simulink model "B4_quadcopter_model_discrete"  (R2021b)
settings: Solver=VariableStepAuto  StartTime=0.0  StopTime=10  FixedStep=0.002  RelTol=1e-3
values from neighbouring files (symbols this model uses):
  coef_sim_1 = tf_des_d.Denominator{1}(2)    [A11_setup_script_pprz.m]    (also in A1_setup_script.m; A6_slow_actuator.m)
  coef_sim_2 = tf_des_d.Numerator{1}(2)    [A11_setup_script_pprz.m]    (also in A1_setup_script.m; A6_slow_actuator.m)
  doublet_mag = - 0.15    (= -0.15)    [A11_setup_script_pprz.m]    (also in A1_setup_script.m)
  doublet_time = 6    [A11_setup_script_pprz.m]    (also in A1_setup_script.m)
  f_8 = 1    [A11_setup_script_pprz.m]    (also in A1_setup_script.m)
  FILT_CUTOFF = 2*pi*5    (= 31.4159265359)    [A11_setup_script_pprz.m]    (also in A1_setup_script.m)
  FILTER = 1    [A11_setup_script_pprz.m]    (also in A1_setup_script.m)
  G1 = inv(I)*G1_r    [A10_simple_plant.m]    (also in A11_setup_script_pprz.m = G1/scale; A1_setup_script.m = [G1;G1_T])
  G1_simple = inv(I)*G1_r_simple    [A1_setup_script.m]
  G2 = G2/scale    [A11_setup_script_pprz.m]    (also in A1_setup_script.m = (1/sampling_time)*inv(I)*(G2_r))
  h_plate = 0.3    [A11_setup_script_pprz.m]    (also in A1_setup_script.m = 0.16)
  I = eye(3,3)    [A10_simple_plant.m]    (also in A11_setup_script_pprz.m; A1_setup_script.m; A2_B_matrix_generation_symbolic.m = [Ixx 0 0; A3_B_matrix_generation_symbolic_cascaded.m = [Ixx 0 0)
  Iyy = 0.0008    [A11_setup_script_pprz.m]    (also in A1_setup_script.m = 0.0015)
  Izz = 0.000498    [A11_setup_script_pprz.m]    (also in A1_setup_script.m = 0.00015)
  K = 7    [A11_setup_script_pprz.m]    (also in A1_setup_script.m = 10)
  K_act = 50    [A10_simple_plant.m]    (also in A11_setup_script_pprz.m = 20; A1_setup_script.m = 20)
  K_act_outer = diag([K K K_act])    [A1_setup_script.m]
  K_d = 15    [A11_setup_script_pprz.m]    (also in A1_setup_script.m = 25)
  K_dd = K_act    (= 20)    [A11_setup_script_pprz.m]    (also in A1_setup_script.m)
  K_dyn = K    (= 10)    [A1_setup_script.m]
  K_ec = 50    [A11_setup_script_pprz.m]    (also in A1_setup_script.m = 251)
  K_ec_d = 13    [A11_setup_script_pprz.m]    (also in A1_setup_script.m = 25)
  K_ec_d_u = 1.5    [A11_setup_script_pprz.m]    (also in A1_setup_script.m = 5)
  K_ec_d_v = 1.5    [A11_setup_script_pprz.m]    (also in A1_setup_script.m = 5)
  K_ec_d_w = 1.5    [A11_setup_script_pprz.m]    (also in A1_setup_script.m = 5)
  K_ec_dd = 9    [A11_setup_script_pprz.m]    (also in A1_setup_script.m = 45)
  K_ec_i = 0    [A11_setup_script_pprz.m]    (also in A1_setup_script.m = 380)
  K_ec_u = 1.5    [A11_setup_script_pprz.m]    (also in A1_setup_script.m = 5)
  K_ec_v = 1.5    [A11_setup_script_pprz.m]    (also in A1_setup_script.m = 5)
  K_ec_w = 1.5    [A11_setup_script_pprz.m]    (also in A1_setup_script.m = 5)
  K_t = 0.0005    [A10_simple_plant.m]    (also in A11_setup_script_pprz.m = 6.557e-08; A1_setup_script.m = 6.557e-08)
  K_u = 1.0    (= 1)    [A11_setup_script_pprz.m]    (also in A1_setup_script.m = 1.5)
  K_u_d = 2.5    [A11_setup_script_pprz.m]    (also in A1_setup_script.m = 7)
  K_u_dd = K    (= 10)    [A1_setup_script.m]
  K_v = 1.0    (= 1)    [A11_setup_script_pprz.m]    (also in A1_setup_script.m = 1.5)
  K_v_d = 2.5    [A11_setup_script_pprz.m]    (also in A1_setup_script.m = 7)
  K_v_dd = K    (= 10)    [A1_setup_script.m]
  K_w = 1.0    (= 1)    [A11_setup_script_pprz.m]    (also in A1_setup_script.m = 4.5)
  K_w_d = 2.5    [A11_setup_script_pprz.m]    (also in A1_setup_script.m = 7)
  K_w_dd = K    (= 10)    [A1_setup_script.m]
  l_plate = 0.1    [A11_setup_script_pprz.m]    (also in A1_setup_script.m = 0.11)
  m = 0.4    [A10_simple_plant.m]    (also in A11_setup_script_pprz.m; A1_setup_script.m)
  NOISE = 0    [A11_setup_script_pprz.m]    (also in A1_setup_script.m)
  NOISE_ACC = 0.00005    (= 5e-05)    [A11_setup_script_pprz.m]    (also in A1_setup_script.m)
  NOISE_GYRO = 0.00005    (= 5e-05)    [A11_setup_script_pprz.m]    (also in A1_setup_script.m)
  NOISE_RPM = 200    [A11_setup_script_pprz.m]    (also in A1_setup_script.m)
  omega_act = 50    [A6_slow_actuator.m]
  omega_des = 20.00    (= 20)    [A11_setup_script_pprz.m]    (also in A1_setup_script.m; A6_slow_actuator.m = 49)
  sampling_time = 1/frequency    (= 0.002)    [A11_setup_script_pprz.m]    (also in A12_sim_multi_run.m; A1_setup_script.m; A6_slow_actuator.m)
  scale_8 = 1.6    [A11_setup_script_pprz.m]    (also in A1_setup_script.m)
  start_8 = 2    [A11_setup_script_pprz.m]    (also in A1_setup_script.m)
  start_time = 2    [A11_setup_script_pprz.m]    (also in A1_setup_script.m = 1)
  t_8 = 10    [A11_setup_script_pprz.m]    (also in A1_setup_script.m)
  w_plate = 0.3    [A11_setup_script_pprz.m]    (also in A1_setup_script.m = 0.36)
undefined symbols (not defined in the file or in its folder): DiscIntNeverNeededParam, K_ec_d_p, K_ec_d_q, K_ec_d_r, K_ec_dd_p, K_ec_dd_q, K_ec_dd_r, K_ec_i_u, K_ec_i_v, K_ec_i_w, K_ec_p, K_ec_q, K_ec_r, K_p, K_p_d, K_p_dd, K_q, K_q_d, K_q_dd, K_r, K_r_d, K_r_dd
libraries: simulink x44, cstblocks x37, dspinverses x26, dspmathops x9, dspstat3 x9, aerolibutil x9, sharedutil x3, aerolibanim x1
(part 7 of 13)

== system B4_quadcopter_model_discrete/Discrete Model - Complementary Filtering/Discrete INDI Controller Cascaded w// Actuator Compensation/ERROR CONTROLLER VELOCITY ==
  Vx_ref : Inport
  Vy_ref : Inport  Port=2
  Vz_ref : Inport  Port=3
  X_ref : Inport  Port=4
  Y_ref : Inport  Port=5
  Z_ref : Inport  Port=6
  Gain : Gain  Gain=K_ec_u
  Gain1 : Gain  Gain=K_ec_d_u
  Gain2 : Gain  Gain=K_ec_v
  Gain3 : Gain  Gain=K_ec_d_v
  Gain4 : Gain  Gain=K_ec_v
  Gain5 : Gain  Gain=K_ec_d_v
  Sum{,3,5..8} (6 alike) : Sum  Inputs=|+-
  Sum1 : Sum  Inputs=|++
  Sum2 : Sum  Inputs=|++
  Sum4 : Sum  Inputs=|++
  Ax_ec : Outport
  Ay_ec : Outport  Port=2
  Az_ec : Outport  Port=3
  wires:
  [Vz] -> Sum6/2
  Sum1/1 -> Ax_ec/1
  Sum2/1 -> Ay_ec/1
  Vy_ref/1 -> Sum3/1
  Vx_ref/1 -> Sum/1
  [Vy] -> Sum3/2
  Vz_ref/1 -> Sum6/1
  Sum/1 -> Gain1/1  "Vx_error"
  Sum4/1 -> Az_ec/1
  [Vx] -> Sum/2
  [x] -> Sum5/2
  X_ref/1 -> Sum5/1
  Sum5/1 -> Gain/1
  Gain1/1 -> Sum1/1
  Gain/1 -> Sum1/2
  Gain3/1 -> Sum2/1
  Sum3/1 -> Gain3/1  "Vy_error"
  Gain5/1 -> Sum4/1
  Sum6/1 -> Gain5/1  "Vz_error"
  Y_ref/1 -> Sum7/1
  [y] -> Sum7/2
  Sum7/1 -> Gain2/1
  Z_ref/1 -> Sum8/1
  [z] -> Sum8/2
  Sum8/1 -> Gain4/1
  Gain4/1 -> Sum4/2
  Gain2/1 -> Sum2/2

== system B4_quadcopter_model_discrete/Discrete Model - Complementary Filtering/Discrete INDI Controller Cascaded w// Actuator Compensation/INTERNAL REFERENCE MODEL ATTITUDE ==
  phi_cmd : Inport
  theta_cmd : Inport  Port=2
  psi_cmd : Inport  Port=3
  Discrete-Time Integrator{,1..8} (9 alike) : DiscreteIntegrator  SampleTime=sampling_time  ICPrevOutput=DiscIntNeverNeededParam  ICPrevScaledInput=DiscIntNeverNeededParam
  Gain1 : Gain  Gain=K
  Gain2 : Gain  Gain=K_dd
  Gain3 : Gain  Gain=K
  Gain4 : Gain  Gain=K_d
  Gain5 : Gain  Gain=K_d
  Gain6 : Gain  Gain=K_d
  Gain7 : Gain  Gain=K
  Gain8 : Gain  Gain=K_dd
  Gain9 : Gain  Gain=K_dd
  MATLAB Function1 : MATLAB Function  TreatAsAtomicUnit=on
  Scope : Scope  NumInputPorts=2
  Sum{1..4,11,16,20..22} (9 alike) : Sum  Inputs=|+-
  body rates to euler rates : Subsystem
  euler rates to body rates : Subsystem
  pdd_ref : Outport
  qdd_ref : Outport  Port=2
  rdd_ref : Outport  Port=3
  pd_ref : Outport  Port=4
  qd_ref : Outport  Port=5
  rd_ref : Outport  Port=6
  p_ref : Outport  Port=7
  q_ref : Outport  Port=8
  r_ref : Outport  Port=9
  phi_ref : Outport  Port=10
  theta_ref : Outport  Port=11
  psi_ref : Outport  Port=12
  tag scope: p_ref=global, phi_ref=global, psi_ref=global, q_ref=global, r_ref=global, theta_ref=global
  wires:
  Discrete-Time Integrator1/1 -> [theta_ref], theta_ref/1, Sum11/2  "theta_ref"
  Discrete-Time Integrator8/1 -> Sum4/2, Discrete-Time Integrator5/1, rd_ref/1  "rd_ref"
  Discrete-Time Integrator3/1 -> [p_ref], p_ref/1, body rates to euler rates/1(p), Sum21/2  "p_ref"
  Discrete-Time Integrator5/1 -> [r_ref], r_ref/1, body rates to euler rates/3(r), Sum22/2  "r_ref"
  Discrete-Time Integrator4/1 -> Scope/1, body rates to euler rates/2(q), [q_ref], q_ref/1, Sum16/2  "q_ref"
  Discrete-Time Integrator7/1 -> Sum3/2, Discrete-Time Integrator4/1, qd_ref/1  "qd_ref"
  Sum21/1 -> Gain4/1
  Sum11/1 -> Gain1/1
  Sum22/1 -> Gain6/1
  Sum16/1 -> Gain5/1
  Discrete-Time Integrator2/1 -> [phi_ref], phi_ref/1, Sum20/2  "phi_ref"
  Sum20/1 -> Gain7/1
  Discrete-Time Integrator6/1 -> Sum2/2, Discrete-Time Integrator3/1, pd_ref/1  "pd_ref"
  phi_cmd/1 -> Sum20/1  "phi_cmd"
  theta_cmd/1 -> Sum11/1  "theta_cmd"
  psi_cmd/1 -> Sum1/1  "psi_cmd"
  Discrete-Time Integrator/1 -> [psi_ref], psi_ref/1, Sum1/2  "psi_ref"
  Sum1/1 -> MATLAB Function1/1(pis_e)  "err"
  Gain4/1 -> Sum2/1
  Gain5/1 -> Sum3/1
  Gain6/1 -> Sum4/1
  Sum2/1 -> Gain2/1
  Sum3/1 -> Gain8/1
  Sum4/1 -> Gain9/1
  Gain2/1 -> Discrete-Time Integrator6/1, pdd_ref/1  "pdd_ref"
  Gain8/1 -> Discrete-Time Integrator7/1, qdd_ref/1  "qdd_ref"
  Gain9/1 -> Discrete-Time Integrator8/1, rdd_ref/1  "rdd_ref"
  Gain7/1 -> euler rates to body rates/1(phi_dot)
  euler rates to body rates/1(p) -> Sum21/1
  Gain1/1 -> euler rates to body rates/2(theta_dot)
  euler rates to body rates/2(q) -> Sum16/1
  Gain3/1 -> euler rates to body rates/3(psi_dot)
  euler rates to body rates/3(r) -> Sum22/1
  body rates to euler rates/3(psi_dot) -> Discrete-Time Integrator/1
  body rates to euler rates/2(theta_dot) -> Scope/2, Discrete-Time Integrator1/1
  body rates to euler rates/1(phi_dot) -> Discrete-Time Integrator2/1
  MATLAB Function1/1(psie_w) -> Gain3/1  "wrapped_Err"

== system B4_quadcopter_model_discrete/Discrete Model - Complementary Filtering/Discrete INDI Controller Cascaded w// Actuator Compensation/INTERNAL REFERENCE MODEL VELOCITY ==
  Vx_cmd : Inport
  Vy_cmd : Inport  Port=2
  Vz_cmd : Inport  Port=3
  Discrete-Time Integrator{,1..5} (6 alike) : DiscreteIntegrator  SampleTime=-1  ICPrevOutput=DiscIntNeverNeededParam  ICPrevScaledInput=DiscIntNeverNeededParam
  Gain1 : Gain  Gain=K_w_d
  Gain2 : Gain  Gain=K_v_d
  Gain3 : Gain  Gain=K_w
  Gain4 : Gain  Gain=K_v
  Gain5 : Gain  Gain=K_u
  Gain9 : Gain  Gain=K_u_d
  Sum{1..4,11,20} (6 alike) : Sum  Inputs=|+-
  Ax_ref : Outport
  Ay_ref : Outport  Port=2
  Az_ref : Outport  Port=3
  Vx_ref : Outport  Port=4
  Vy_ref : Outport  Port=5
  Vz_ref : Outport  Port=6
  X_ref : Outport  Port=7
  Y_ref : Outport  Port=8
  Z_ref : Outport  Port=9
  tag scope: Ax_ref=global, Ay_ref=global, Az_ref=global, Vx_ref=global, Vy_ref=global, Vz_ref=global
  wires:
  Discrete-Time Integrator1/1 -> Sum3/2, Discrete-Time Integrator4/1, [Vy_ref], Vz_ref/1
  Gain1/1 -> Discrete-Time Integrator1/1, [Az_ref], Az_ref/1
  Gain9/1 -> Discrete-Time Integrator/1, [Ax_ref], Ax_ref/1
  Vy_cmd/1 -> Sum1/1
  Discrete-Time Integrator/1 -> Sum4/2, Discrete-Time Integrator3/1, [Vx_ref], Vx_ref/1
  Vx_cmd/1 -> Sum20/1
  Vz_cmd/1 -> Sum11/1
  Discrete-Time Integrator2/1 -> Sum2/2, Discrete-Time Integrator5/1, [Vz_ref], Vy_ref/1
  Gain2/1 -> Discrete-Time Integrator2/1, [Ay_ref], Ay_ref/1
  Sum20/1 -> Gain5/1
  Sum11/1 -> Gain3/1
  Sum1/1 -> Gain4/1
  Gain4/1 -> Sum2/1
  Gain3/1 -> Sum3/1
  Gain5/1 -> Sum4/1
  Sum3/1 -> Gain1/1
  Sum2/1 -> Gain2/1
  Sum4/1 -> Gain9/1
  Discrete-Time Integrator3/1 -> X_ref/1, Sum20/2
  Discrete-Time Integrator4/1 -> Sum11/2, Z_ref/1
  Discrete-Time Integrator5/1 -> Sum1/2, Y_ref/1

== system B4_quadcopter_model_discrete/Discrete Model - Complementary Filtering/Discrete INDI Controller Cascaded w// Actuator Compensation/Subsystem ==
  Constant : Constant  Value=w_plate
  Constant1 : Constant  Value=Iyy
  Constant10 : Constant  Value=l_plate
  Constant11 : Constant  Value=h_plate
  Constant2 : Constant  Value=l_plate
  Constant3 : Constant  Value=h_plate
  Constant4 : Constant  Value=w_plate
  Constant5 : Constant  Value=Izz
  Constant6 : Constant  Value=l_plate
  Constant7 : Constant  Value=h_plate
  Constant8 : Constant  Value=w_plate
  Constant9 : Constant  Value=Izz
  MATLAB Function : MATLAB Function  TreatAsAtomicUnit=on
  MATLAB Function1 : MATLAB Function  TreatAsAtomicUnit=on
  MATLAB Function2 : MATLAB Function  TreatAsAtomicUnit=on
  Terminator{,1..5} (6 alike) : Terminator
  body rates to euler rates : Subsystem
  body rates to euler rates1 : Subsystem
  body rates to euler rates2 : Subsystem
  qdd_comp : Outport
  rdd_comp1 : Outport  Port=2
  rdd_comp : Outport  Port=3
  wires:
  MATLAB Function/1(qdd_comp) -> qdd_comp/1  "qdd_comp"
  [theta] -> MATLAB Function/1(theta)
  [Vx] -> MATLAB Function/3(Vx)
  [Ax] -> MATLAB Function/5(Ax)
  Constant/1 -> MATLAB Function/7(w_plate)
  Constant1/1 -> MATLAB Function/10(Iyy)
  Constant2/1 -> MATLAB Function/9(l_plate)
  Constant3/1 -> MATLAB Function/8(h_plate)
  [p] -> body rates to euler rates/1(p)
  [q] -> body rates to euler rates/2(q)
  [r] -> body rates to euler rates/3(r)
  body rates to euler rates/2(theta_dot) -> MATLAB Function/2(dtheta)
  body rates to euler rates/1(phi_dot) -> Terminator/1
  [Vy] -> MATLAB Function/4(Vy)
  [Ay] -> MATLAB Function/6(Ay)
  body rates to euler rates/3(psi_dot) -> Terminator1/1
  [theta] -> MATLAB Function1/1(theta)
  [p] -> body rates to euler rates1/1(p)
  Constant7/1 -> MATLAB Function1/8(h_plate)
  [Ax] -> MATLAB Function1/5(Ax)
  [q] -> body rates to euler rates1/2(q)
  [Vx] -> MATLAB Function1/3(Vx)
  Constant6/1 -> MATLAB Function1/9(l_plate)
  MATLAB Function1/1(rdd_comp) -> rdd_comp/1  "rdd_comp"
  [Vy] -> MATLAB Function1/4(Vy)
  [r] -> body rates to euler rates1/3(r)
  body rates to euler rates1/2(theta_dot) -> MATLAB Function1/2(dtheta)
  Constant4/1 -> MATLAB Function1/7(w_plate)
  body rates to euler rates1/1(phi_dot) -> Terminator2/1
  Constant5/1 -> MATLAB Function1/10(Izz)
  [Ay] -> MATLAB Function1/6(Ay)
  body rates to euler rates1/3(psi_dot) -> Terminator3/1
  body rates to euler rates2/2(theta_dot) -> MATLAB Function2/2(dtheta)
  Constant8/1 -> MATLAB Function2/7(w_plate)
  body rates to euler rates2/3(psi_dot) -> Terminator5/1
  [Vy_ref] -> MATLAB Function2/4(Vy)
  Constant9/1 -> MATLAB Function2/10(Izz)
  [Ax_ref] -> MATLAB Function2/5(Ax)
  body rates to euler rates2/1(phi_dot) -> Terminator4/1
  [Ay_ref] -> MATLAB Function2/6(Ay)
  [q_ref] -> body rates to euler rates2/2(q)
  [r_ref] -> body rates to euler rates2/3(r)
  MATLAB Function2/1(rdd_comp) -> rdd_comp1/1  "rdd_comp_ref"
  [p_ref] -> body rates to euler rates2/1(p)
  Constant10/1 -> MATLAB Function2/9(l_plate)
  Constant11/1 -> MATLAB Function2/8(h_plate)
  [theta_ref] -> MATLAB Function2/1(theta)
  [Vx_ref] -> MATLAB Function2/3(Vx)

== system B4_quadcopter_model_discrete/Discrete Model - Complementary Filtering/Discrete INDI Controller Cascaded w// Actuator Compensation Double/8-shape trajectory ==
  Clock : Clock
      settings: Decimation=100
  Constant : Constant  Value=f_8
  Constant1 : Constant  Value=scale_8
  Constant2 : Constant  Value=t_8
  Constant3 : Constant  Value=sampling_time
  Constant4 : Constant  Value=0
  Constant5 : Constant  Value=start_8
  Constant6 : Constant  Value=t_8
  Constant7 : Constant  Value=start_8
  Discrete Derivative : simulink/Discrete/Discrete Derivative  gainval=1.0  ICPrevScaledInput=0.0  OutMin=[]  OutMax=[]  OutDataType=fixdt(1, 16)  OutScaling=2^-10  DoSatur=off
  Discrete Derivative1 : simulink/Discrete/Discrete Derivative  gainval=1.0  ICPrevScaledInput=0.0  OutMin=[]  OutMax=[]  OutDataType=fixdt(1, 16)  OutScaling=2^-10  DoSatur=off
  MATLAB Function : MATLAB Function  TreatAsAtomicUnit=on
  Scope : Scope
  Sum : Sum  Inputs=|+-
  Sum3 : Sum  Inputs=|+-
  Sum7 : Sum  Inputs=|+-
  Switch : Switch  Criteria=u2 > Threshold  Threshold=t_8
  Switch1 : Switch  Criteria=u2 > Threshold  Threshold=start_8
  Zero-Order Hold : ZeroOrderHold  SampleTime=sampling_time
  xd_traj : Outport
  yd_traj : Outport  Port=2
  psi_traj : Outport  Port=3
  wires:
  Constant2/1 -> Switch/1
  Switch/1 -> Scope/1, MATLAB Function/1(t)  "t"
  Constant/1 -> MATLAB Function/2(f)
  MATLAB Function/2(y) -> Sum7/2, Discrete Derivative1/1  "y_traj"
  Zero-Order Hold/1 -> Switch/2, Switch/3
  Constant1/1 -> MATLAB Function/3(scale)
  Constant3/1 -> MATLAB Function/4(sampling_time)
  MATLAB Function/1(x) -> Discrete Derivative/1, Sum3/2  "x_traj"
  MATLAB Function/3(psi) -> psi_traj/1  "psi_traj"
  Discrete Derivative/1 -> xd_traj/1  "xd_traj"
  Discrete Derivative1/1 -> yd_traj/1  "yd_traj"
  Clock/1 -> Sum/1, Switch1/2
  Constant4/1 -> Switch1/3
  Switch1/1 -> Zero-Order Hold/1
  Constant5/1 -> Sum/2
  Sum/1 -> Switch1/1
  Constant6/1 -> MATLAB Function/5(total_time)
  Sum7/1 -> ?
  ? -> ?
  ? -> ?
  [y] -> Sum7/1
  ? -> ?
  ? -> ?  "pos_err"
  [x] -> Sum3/1
  Sum3/1 -> ?
  Constant7/1 -> MATLAB Function/6(start_time)

== system B4_quadcopter_model_discrete/Discrete Model - Complementary Filtering/Discrete INDI Controller Cascaded w// Actuator Compensation Double/Butterworth Lowpass 2nd Order3 ==
  In : Inport
  Constant : Constant  Value=FILTER  SampleTime=sampling_time
  Merge : Merge
  Switch Case : SwitchCase
  Switch Case Action Subsystem : Subsystem  TreatAsAtomicUnit=on
  Switch Case Action Subsystem1 : Subsystem  TreatAsAtomicUnit=on
  psi_cmd : Outport
  wires:
  Merge/1 -> psi_cmd/1
  Switch Case Action Subsystem/1(Out1) -> Merge/1
  Constant/1 -> Switch Case/1
  Switch Case Action Subsystem1/1(Out1) -> Merge/2
  Switch Case/2 -> Switch Case Action Subsystem1/Action
  In/1 -> Switch Case Action Subsystem/1(In1), Switch Case Action Subsystem1/1(In1)
  Switch Case/1 -> Switch Case Action Subsystem/Action

== system B4_quadcopter_model_discrete/Discrete Model - Complementary Filtering/Discrete INDI Controller Cascaded w// Actuator Compensation Double/Doublet Block ==
  Scope : Scope
  Step : Step  Time=start_time  After=doublet_mag  SampleTime=sampling_time
  Step1 : Step  Time=start_time + doublet_time/2  After=-doublet_mag*2  SampleTime=sampling_time
  Step2 : Step  Time=start_time + doublet_time  After=doublet_mag  SampleTime=sampling_time
  Sum : Sum  Inputs=|++
  Sum1 : Sum  Inputs=|++
  Out1 : Outport
  wires:
  Step/1 -> Sum/1
  Step1/1 -> Sum/2
  Sum/1 -> Sum1/1
  Sum1/1 -> Out1/1, Scope/1
  Step2/1 -> Sum1/2

== system B4_quadcopter_model_discrete/Discrete Model - Complementary Filtering/Discrete INDI Controller Cascaded w// Actuator Compensation Double/Drag Plate Aerodynamics ==
  Constant : Constant  Value=0
  Constant2 : Constant  Value=w_plate
  Constant3 : Constant  Value=h_plate
  Constant5 : Constant  Value=l_plate
  Mux : Mux  Inputs=3
  Terminator : Terminator
  Terminator1 : Terminator
  drag plate My : MATLAB Function  TreatAsAtomicUnit=on
  Aero Moment : Outport
  Fx_earth : Outport  Port=2
  wires:
  Mux/1 -> Aero Moment/1  "aero_moment"
  Constant/1 -> Mux/3, Mux/1
  drag plate My/1(My_dp) -> Mux/2  "My_dp"
  Constant2/1 -> drag plate My/1(w_plate)
  Constant3/1 -> drag plate My/2(h_plate)
  Constant5/1 -> drag plate My/3(l_plate)
  [theta_cont] -> drag plate My/4(theta)
  drag plate My/4(Cl) -> Terminator/1  "Cl"
  drag plate My/5(Cd) -> Terminator1/1  "Cd"
  [Vx_cont] -> drag plate My/5(Vx)
  drag plate My/2(Fx_earth) -> Fx_earth/1  "Fx_aero_earth"

== system B4_quadcopter_model_discrete/Discrete Model - Complementary Filtering/Discrete INDI Controller Cascaded w// Actuator Compensation Double/ERROR CONTROLLER ATTITUDE ==
  pd_ref : Inport
  qd_ref : Inport  Port=2
  rd_ref : Inport  Port=3
  p_ref : Inport  Port=4
  q_ref : Inport  Port=5
  r_ref : Inport  Port=6
  phi_ref : Inport  Port=7
  theta_ref : Inport  Port=8
  psi_ref : Inport  Port=9
  Add : Sum  Inputs=+++
  Add1 : Sum  Inputs=+++
  Add2 : Sum  Inputs=+++
  Gain : Gain  Gain=K_ec_dd_p + K_act
  Gain1 : Gain  Gain=K_ec_d_p *(1 + K_act)
  Gain2 : Gain  Gain=K_ec_p *(1 + K_act)
  Gain3 : Gain  Gain=K_ec_dd_q + K_act
  Gain4 : Gain  Gain=K_ec_d_q *(1 + K_act)
  Gain5 : Gain  Gain=K_ec_q *(1 + K_act)
  Gain6 : Gain  Gain=K_ec_dd_r + K_act
  Gain7 : Gain  Gain=K_ec_d_r *(1 + K_act)
  Gain8 : Gain  Gain=K_ec_r *(1 + K_act)
  Sum{,1..8} (9 alike) : Sum  Inputs=|+-
  pdd_ec : Outport
  qdd_ec : Outport  Port=2
  rdd_ec : Outport  Port=3
  wires:
  pd_ref/1 -> Sum/1
  p_ref/1 -> Sum1/1
  Add/1 -> pdd_ec/1
  [p] -> Sum1/2
  [phi] -> Sum2/2
  phi_ref/1 -> Sum2/1
  [pd_f] -> Sum/2
  Sum/1 -> Gain/1  "pd_err"
  Gain/1 -> Add/1
  Sum1/1 -> Gain1/1  "p_err"
  Sum2/1 -> Gain2/1  "phi_err"
  Gain1/1 -> Add/2
  Gain2/1 -> Add/3
  Sum4/1 -> Gain4/1  "q_err"
  [qd_f] -> Sum3/2
  Gain4/1 -> Add1/2
  Gain5/1 -> Add1/3
  theta_ref/1 -> Sum5/1
  [theta] -> Sum5/2
  [q] -> Sum4/2
  Gain3/1 -> Add1/1
  q_ref/1 -> Sum4/1
  Add1/1 -> qdd_ec/1
  qd_ref/1 -> Sum3/1
  Sum7/1 -> Gain7/1  "r_err"
  Sum8/1 -> Gain8/1  "psi_err"
  Sum6/1 -> Gain6/1  "rd_err"
  [rd_f] -> Sum6/2
  Gain7/1 -> Add2/2
  Gain8/1 -> Add2/3
  psi_ref/1 -> Sum8/1
  [psi] -> Sum8/2
  [r] -> Sum7/2
  Gain6/1 -> Add2/1
  r_ref/1 -> Sum7/1
  Add2/1 -> rdd_ec/1
  rd_ref/1 -> Sum6/1
  Sum3/1 -> Gain3/1  "qd_err"
  Sum5/1 -> Gain5/1  "theta_err"

== system B4_quadcopter_model_discrete/Discrete Model - Complementary Filtering/Discrete INDI Controller Cascaded w// Actuator Compensation Double/ERROR CONTROLLER VELOCITY ==
  Ax_ref : Inport
  Ay_ref : Inport  Port=2
  Az_ref : Inport  Port=3
  Vx_ref : Inport  Port=4
  Vy_ref : Inport  Port=5
  Vz_ref : Inport  Port=6
  Add1 : Sum  Inputs=+++
  Add2 : Sum  Inputs=+++
  Add3 : Sum  Inputs=+++
  Discrete-Time Integrator : DiscreteIntegrator  SampleTime=-1  ICPrevOutput=DiscIntNeverNeededParam  ICPrevScaledInput=DiscIntNeverNeededParam
  Discrete-Time Integrator1 : DiscreteIntegrator  SampleTime=-1  ICPrevOutput=DiscIntNeverNeededParam  ICPrevScaledInput=DiscIntNeverNeededParam
  Discrete-Time Integrator2 : DiscreteIntegrator  SampleTime=-1  ICPrevOutput=DiscIntNeverNeededParam  ICPrevScaledInput=DiscIntNeverNeededParam
  Gain : Gain  Gain=K_ec_d_w + K_dyn
  Gain2 : Gain  Gain=K_ec_d_v + K_dyn
  Gain3 : Gain  Gain=K_ec_i_v *(1 + K_dyn)
  Gain4 : Gain  Gain=K_ec_w *(1 + K_dyn)
  Gain5 : Gain  Gain=K_ec_v *(1 + K_dyn)
  Gain6 : Gain  Gain=K_ec_d_u + K_dyn
  Gain7 : Gain  Gain=K_ec_i_u *(1 + K_dyn)
  Gain8 : Gain  Gain=K_ec_u *(1 + K_dyn)
  Gain9 : Gain  Gain=K_ec_i_w *(1 + K_dyn)
  Sum{1..6} (6 alike) : Sum  Inputs=|+-
  Jx_ec : Outport
  Jy_ec : Outport  Port=2
  Jz_ec : Outport  Port=3
  wires:
  [Vz] -> Sum6/2
  Discrete-Time Integrator/1 -> Gain9/1
  Sum6/1 -> Discrete-Time Integrator/1, Gain4/1  "Vz_error"
  Vz_ref/1 -> Sum6/1
  Az_ref/1 -> Sum5/1
  [Az_f] -> Sum5/2
  Gain4/1 -> Add1/2
  Gain9/1 -> Add1/3
  Add1/1 -> Jz_ec/1
  Sum5/1 -> Gain/1
  Gain/1 -> Add1/1
  Add2/1 -> Jy_ec/1
  Ay_ref/1 -> Sum1/1
  Gain5/1 -> Add2/2
  Gain3/1 -> Add2/3
  Gain2/1 -> Add2/1
  Sum1/1 -> Gain2/1
  [Ay_f] -> Sum1/2
  Vy_ref/1 -> Sum2/1
  Sum2/1 -> Discrete-Time Integrator1/1, Gain5/1  "Vy_error"
  [Vy] -> Sum2/2
  Discrete-Time Integrator1/1 -> Gain3/1
  [Vx] -> Sum4/2
  Sum4/1 -> Discrete-Time Integrator2/1, Gain8/1  "Vx_error"
  Discrete-Time Integrator2/1 -> Gain7/1
  Gain8/1 -> Add3/2
  [Ax_f] -> Sum3/2
  Sum3/1 -> Gain6/1
  Gain7/1 -> Add3/3
  Ax_ref/1 -> Sum3/1
  Vx_ref/1 -> Sum4/1
  Gain6/1 -> Add3/1
  Add3/1 -> Jx_ec/1

== system B4_quadcopter_model_discrete/Discrete Model - Complementary Filtering/Discrete INDI Controller Cascaded w// Actuator Compensation Double/INTERNAL REFERENCE MODEL ATTITUDE ==
  phi_cmd : Inport
  theta_cmd : Inport  Port=2
  psi_cmd : Inport  Port=3
  Discrete-Time Integrator{,1..8} (9 alike) : DiscreteIntegrator  SampleTime=sampling_time  ICPrevOutput=DiscIntNeverNeededParam  ICPrevScaledInput=DiscIntNeverNeededParam
  Gain1 : Gain  Gain=K_q_dd
  Gain2 : Gain  Gain=K_p_dd
  Gain3 : Gain  Gain=K_r_dd
  Gain4 : Gain  Gain=K_p_d
  Gain5 : Gain  Gain=K_q_d
  Gain6 : Gain  Gain=K_r_d
  Gain7 : Gain  Gain=K_p
  Gain8 : Gain  Gain=K_q
  Gain9 : Gain  Gain=K_r
  Scope : Scope  NumInputPorts=2
  Sum{1..4,11,16,20..22} (9 alike) : Sum  Inputs=|+-
  body rates to euler rates : Subsystem
  euler rates to body rates : Subsystem
  pdd_ref : Outport
  qdd_ref : Outport  Port=2
  rdd_ref : Outport  Port=3
  pd_ref : Outport  Port=4
  qd_ref : Outport  Port=5
  rd_ref : Outport  Port=6
  p_ref : Outport  Port=7
  q_ref : Outport  Port=8
  r_ref : Outport  Port=9
  phi_ref : Outport  Port=10
  theta_ref : Outport  Port=11
  psi_ref : Outport  Port=12
  tag scope: p_ref=global, phi_ref=global, psi_ref=global, q_ref=global, r_ref=global, theta_ref=global
  wires:
  Discrete-Time Integrator1/1 -> [theta_ref], theta_ref/1, Sum11/2  "theta_ref"
  Discrete-Time Integrator8/1 -> Sum4/2, Discrete-Time Integrator5/1, rd_ref/1  "rd_ref"
  Discrete-Time Integrator3/1 -> [p_ref], p_ref/1, body rates to euler rates/1(p), Sum21/2  "p_ref"
  Discrete-Time Integrator5/1 -> [r_ref], r_ref/1, body rates to euler rates/3(r), Sum22/2  "r_ref"
  Discrete-Time Integrator4/1 -> Scope/1, body rates to euler rates/2(q), [q_ref], q_ref/1, Sum16/2  "q_ref"
  Discrete-Time Integrator7/1 -> Sum3/2, Discrete-Time Integrator4/1, qd_ref/1  "qd_ref"
  Sum21/1 -> Gain4/1
  Sum11/1 -> Gain8/1
  Sum22/1 -> Gain6/1
  Sum16/1 -> Gain5/1
  Discrete-Time Integrator2/1 -> [phi_ref], phi_ref/1, Sum20/2  "phi_ref"
  Sum20/1 -> Gain7/1
  Discrete-Time Integrator6/1 -> Sum2/2, Discrete-Time Integrator3/1, pd_ref/1  "pd_ref"
  phi_cmd/1 -> Sum20/1
  theta_cmd/1 -> Sum11/1
  psi_cmd/1 -> Sum1/1
  Discrete-Time Integrator/1 -> [psi_ref], psi_ref/1, Sum1/2  "psi_ref"
  Sum1/1 -> Gain9/1
  Gain4/1 -> Sum2/1
  Gain5/1 -> Sum3/1
  Gain6/1 -> Sum4/1
  Sum2/1 -> Gain2/1
  Sum3/1 -> Gain1/1
  Sum4/1 -> Gain3/1
  Gain2/1 -> Discrete-Time Integrator6/1, pdd_ref/1  "pdd_ref"
  Gain1/1 -> Discrete-Time Integrator7/1, qdd_ref/1  "qdd_ref"
  Gain3/1 -> Discrete-Time Integrator8/1, rdd_ref/1  "rdd_ref"
  Gain7/1 -> euler rates to body rates/1(phi_dot)
  euler rates to body rates/1(p) -> Sum21/1
  Gain8/1 -> euler rates to body rates/2(theta_dot)
  euler rates to body rates/2(q) -> Sum16/1
  Gain9/1 -> euler rates to body rates/3(psi_dot)
  euler rates to body rates/3(r) -> Sum22/1
  body rates to euler rates/3(psi_dot) -> Discrete-Time Integrator/1
  body rates to euler rates/2(theta_dot) -> Scope/2, Discrete-Time Integrator1/1
  body rates to euler rates/1(phi_dot) -> Discrete-Time Integrator2/1

== system B4_quadcopter_model_discrete/Discrete Model - Complementary Filtering/Discrete INDI Controller Cascaded w// Actuator Compensation Double/INTERNAL REFERENCE MODEL VELOCITY ==
  Vx_cmd : Inport
  Vy_cmd : Inport  Port=2
  Vz_cmd : Inport  Port=3
  Discrete-Time Integrator{,1..5} (6 alike) : DiscreteIntegrator  SampleTime=-1  ICPrevOutput=DiscIntNeverNeededParam  ICPrevScaledInput=DiscIntNeverNeededParam
  Gain1 : Gain  Gain=K_w_d
  Gain2 : Gain  Gain=K_v_d
  Gain3 : Gain  Gain=K_u_dd
  Gain4 : Gain  Gain=K_w_dd
  Gain5 : Gain  Gain=K_v_dd
  Gain9 : Gain  Gain=K_u_d
  Sum{1..4,11,20} (6 alike) : Sum  Inputs=|+-
  Jx_ref : Outport
  Jy_ref : Outport  Port=2
  Jz_ref : Outport  Port=3
  Ax_ref : Outport  Port=4
  Ay_ref : Outport  Port=5
  Az_ref : Outport  Port=6
  Vx_ref : Outport  Port=7
  Vy_ref : Outport  Port=8
  Vz_ref : Outport  Port=9
  tag scope: Ax_ref=global, Ay_ref=global, Az_ref=global, Jx_ref=global, Jy_ref=global, Jz_ref=global, Vx_ref=global, Vy_ref=global, Vz_ref=global
  wires:
  Discrete-Time Integrator1/1 -> Vz_ref/1, [Vy_ref], Sum11/2
  Gain1/1 -> Sum3/1
  Gain9/1 -> Sum2/1
  Vy_cmd/1 -> Sum1/1
  Discrete-Time Integrator/1 -> [Vx_ref], Vx_ref/1, Sum20/2
  Vx_cmd/1 -> Sum20/1
  Vz_cmd/1 -> Sum11/1
  Discrete-Time Integrator2/1 -> Sum1/2, Vy_ref/1, [Vz_ref]
  Gain2/1 -> Sum4/1
  Sum1/1 -> Gain2/1
  Sum11/1 -> Gain1/1
  Sum20/1 -> Gain9/1
  Gain3/1 -> Jx_ref/1, [Jx_ref], Discrete-Time Integrator3/1
  Gain4/1 -> Jz_ref/1, [Jz_ref], Discrete-Time Integrator4/1
  Gain5/1 -> Jy_ref/1, [Jy_ref], Discrete-Time Integrator5/1
  Sum2/1 -> Gain3/1
  Sum3/1 -> Gain4/1
  Sum4/1 -> Gain5/1
  Discrete-Time Integrator3/1 -> Sum2/2, Ax_ref/1, [Ax_ref], Discrete-Time Integrator/1
  Discrete-Time Integrator4/1 -> Sum3/2, Az_ref/1, [Az_ref], Discrete-Time Integrator1/1
  Discrete-Time Integrator5/1 -> Sum4/2, Ay_ref/1, [Ay_ref], Discrete-Time Integrator2/1

== system B4_quadcopter_model_discrete/Discrete Model - Complementary Filtering/Discrete INDI Controller Cascaded w// Actuator Compensation Double/Pitch Jerk Compensation ==
  Butterworth Lowpass 2nd Order2 : Subsystem
  Constant1 : Constant  Value=Iyy
  Constant2 : Constant  Value=w_plate
  Constant3 : Constant  Value=h_plate
  Constant4 : Constant  Value=l_plate
  Demux : Demux  Outputs=12
  MATLAB Function : MATLAB Function  TreatAsAtomicUnit=on
  Manual Switch : ManualSwitch
  Model Based State Estimate : Subsystem
  Mux1 : Mux  Inputs=12
  State Filtered : Subsystem
  Sum : Sum  Inputs=|+-
  Sum1 : Sum  Inputs=|++
  qdd_comp : Outport
  wires:
  Constant2/1 -> MATLAB Function/13(w_plate)
  Constant3/1 -> MATLAB Function/14(h_plate)
  Constant1/1 -> MATLAB Function/16(Iyy)
  Constant4/1 -> MATLAB Function/15(l_plate)
  MATLAB Function/1(qdd_comp) -> qdd_comp/1
  [psi_ref] -> Mux1/6
  [Ax_ref] -> Mux1/7
  [Vy_ref] -> Mux1/2
  [r_ref] -> Mux1/12
  [phi_ref] -> Mux1/4
  [q_ref] -> Mux1/11
  [Ay_ref] -> Mux1/8
  [theta_ref] -> Mux1/5
  [p_ref] -> Mux1/10
  [Az_ref] -> Mux1/9
  [Vx_ref] -> Mux1/1
  [Vz_ref] -> Mux1/3
  Demux/1 -> MATLAB Function/1(dx)
  Demux/2 -> MATLAB Function/2(dy)
  Demux/3 -> MATLAB Function/3(dz)
  Demux/4 -> MATLAB Function/4(Phi)
  Demux/5 -> MATLAB Function/5(Theta)
  Demux/6 -> MATLAB Function/6(Psi)
  Demux/7 -> MATLAB Function/7(ddx)
  Demux/8 -> MATLAB Function/8(ddy)
  Demux/9 -> MATLAB Function/9(ddz)
  Demux/10 -> MATLAB Function/10(dPhi)
  Demux/11 -> MATLAB Function/11(dTheta)
  Demux/12 -> MATLAB Function/12(dPsi)
  Manual Switch/1 -> Demux/1
  Mux1/1 -> Manual Switch/2  "reference based"
  State Filtered/1(state filtered) -> Sum1/1
  Model Based State Estimate/1(state estimate) -> Sum/1, Butterworth Lowpass 2nd Order2/1(state estimate)
  Butterworth Lowpass 2nd Order2/1(Out) -> Sum/2
  Sum/1 -> ?
  Sum1/1 -> Manual Switch/1

== system B4_quadcopter_model_discrete/Discrete Model - Complementary Filtering/Discrete INDI Controller Cascaded w// Actuator Compensation Double/Pitch Jerk Compensation CopyPaste ==
  Aero Package Easy : Subsystem
  Constant1 : Constant  Value=I  SampleTime=sampling_time
  Demux : Demux  Outputs=3
  Discrete Derivative : simulink/Discrete/Discrete Derivative  gainval=1.0  ICPrevScaledInput=0.0  OutMin=[]  OutMax=[]  OutDataType=fixdt(1, 16)  OutScaling=2^-10  DoSatur=off
  Invert 3x3 Matrix1 : aerolibutil/Invert  3x3 Matrix
  MatrixMultiply : Product  Multiplication=Matrix(*)
  Zero-Order Hold : ZeroOrderHold  SampleTime=sampling_time
  qdd_comp : Outport
  wires:
  Constant1/1 -> Invert 3x3 Matrix1/1
  Aero Package Easy/1(Aero Moment) -> MatrixMultiply/2  "aero_moment"
  Invert 3x3 Matrix1/1 -> MatrixMultiply/1
  Discrete Derivative/1 -> qdd_comp/1
  MatrixMultiply/1 -> Demux/1
  Demux/2 -> Zero-Order Hold/1
  Zero-Order Hold/1 -> Discrete Derivative/1

== system B4_quadcopter_model_discrete/Discrete Model - Complementary Filtering/Discrete INDI Controller Cascaded w// Actuator Compensation Double/Pitch Jerk Compensation1 ==
  Constant2 : Constant  Value=w_plate
  Constant3 : Constant  Value=h_plate
  Constant4 : Constant  Value=m
  MATLAB Function : MATLAB Function  TreatAsAtomicUnit=on
  Terminator : Terminator
  Terminator1 : Terminator
  body rates to euler rates : Subsystem
  Jx_comp : Outport
  wires:
  Constant2/1 -> MATLAB Function/5(w_plate)
  Constant3/1 -> MATLAB Function/6(h_plate)
  Constant4/1 -> MATLAB Function/7(m)
  MATLAB Function/1(Jx_comp) -> Jx_comp/1
  [Ax] -> MATLAB Function/1(Ax)
  [p] -> body rates to euler rates/1(p)
  [q] -> body rates to euler rates/2(q)
  [r] -> body rates to euler rates/3(r)
  body rates to euler rates/1(phi_dot) -> Terminator/1
  body rates to euler rates/3(psi_dot) -> Terminator1/1
  body rates to euler rates/2(theta_dot) -> MATLAB Function/2(dtheta)
  [Vx] -> MATLAB Function/3(Vx)
  [theta] -> MATLAB Function/4(theta)

== system B4_quadcopter_model_discrete/Discrete Model - Complementary Filtering/Force and Moment Calculation/Drag Plate Aerodynamics ==
  Constant : Constant  Value=0
  Constant2 : Constant  Value=w_plate
  Constant3 : Constant  Value=h_plate
  Constant5 : Constant  Value=l_plate
  Mux : Mux  Inputs=3
  Mux1 : Mux  Inputs=3
  Scope : Scope  NumInputPorts=2
  drag plate My : MATLAB Function  TreatAsAtomicUnit=on
  Aero Moment : Outport
  Aero Force : Outport  Port=2
  wires:
  [psi_cont] -> drag plate My/7(heading)
  Mux1/1 -> Aero Force/1  "aero_force"
  drag plate My/3(Fy_earth) -> Mux1/2  "Fy_aero_earth"
  drag plate My/2(Fx_earth) -> Mux1/1  "Fx_aero_earth"
  Constant2/1 -> drag plate My/1(w_plate)
  drag plate My/4(Fz_earth) -> Mux1/3  "Fz_aero_earth"
  Constant3/1 -> drag plate My/2(h_plate)
  Mux/1 -> Aero Moment/1  "aero_moment"
  [Vy_cont] -> drag plate My/6(Vy)
  [theta_cont] -> drag plate My/4(theta)
  [Vx_cont] -> drag plate My/5(Vx)
  Constant5/1 -> drag plate My/3(l_plate)
  Constant/1 -> Mux/2, Mux/1
  drag plate My/1(Mz_dp) -> Mux/3  "Mz_dp"
  [q_cont] -> drag plate My/8(q)
  drag plate My/5(D_plate_vel) -> Scope/1
  drag plate My/6(D_plate_rot) -> Scope/2

== system B4_quadcopter_model_discrete/Discrete Model - Complementary Filtering/Plant and State Estimation/Angular Velocity Model ==
  Constant1 : Constant  Value=sampling_time  SampleTime=sampling_time
  Constant2 : Constant  Value=G1  SampleTime=sampling_time
  Constant3 : Constant  Value=G2  SampleTime=sampling_time
  Constant4 : Constant  Value=I  SampleTime=sampling_time
  Constant5 : Constant  Value=I  SampleTime=sampling_time
  Discrete Derivative : simulink/Discrete/Discrete Derivative  gainval=1.0  ICPrevScaledInput=0.0  OutMin=[]  OutMax=[]  OutDataType=fixdt(1, 16)  OutScaling=2^-10  DoSatur=off
  Drag Plate Aerodynamics : Subsystem
  Gyro : ZeroOrderHold  SampleTime=sampling_time
  Invert 3x3 Matrix1 : aerolibutil/Invert  3x3 Matrix
  Matrix Multiply1 : Product  Multiplication=Matrix(*)
  Moments due to thrust : MATLAB Function  TreatAsAtomicUnit=on
  Sum1 : Sum  Inputs=|++
  Vector Concatenate1 : Concatenate  NumInputs=4
  y_model : Outport
  wires:
  Constant3/1 -> Moments due to thrust/4(G2)
  Constant2/1 -> Moments due to thrust/3(G1)
  Constant1/1 -> Moments due to thrust/5(sampling_time)
  Constant5/1 -> Moments due to thrust/6(I)
  Discrete Derivative/1 -> Moments due to thrust/2(omega_dot)
  Constant4/1 -> Invert 3x3 Matrix1/1
  Invert 3x3 Matrix1/1 -> Matrix Multiply1/1
  Moments due to thrust/1(M_t) -> Sum1/1  "thrust_moment_filter"
  [omega_4_f] -> Vector Concatenate1/4
  [omega_2_f] -> Vector Concatenate1/2
  [omega_1_f] -> Vector Concatenate1/1
  [omega_3_f] -> Vector Concatenate1/3
  Sum1/1 -> Matrix Multiply1/2
  Matrix Multiply1/1 -> y_model/1  "pqr_acc_filter"
  Vector Concatenate1/1 -> Discrete Derivative/1, Moments due to thrust/1(omega)  "actuators"
  Drag Plate Aerodynamics/1(Aero Moment) -> Gyro/1  "aero_moment"
  Gyro/1 -> Sum1/2

== system B4_quadcopter_model_discrete/Discrete Model - Complementary Filtering/Plant and State Estimation/Complementary Filter ==
  y : Inport
  y_model : Inport  Port=2
  Butterworth Lowpass 2nd Order1 : Subsystem
  Butterworth Lowpass 2nd Order2 : Subsystem
  Sum : Sum  Inputs=|++
  Sum1 : Sum  Inputs=|+-
  y_est_no_delay : Outport
  wires:
  y/1 -> Butterworth Lowpass 2nd Order1/1(In)  "y"
  Butterworth Lowpass 2nd Order1/1(Out) -> Sum/1  "y_f"
  Butterworth Lowpass 2nd Order2/1(Out) -> Sum1/2  "y_model_f"
  Sum1/1 -> Sum/2  "y_delay_term"
  y_model/1 -> Butterworth Lowpass 2nd Order2/1(In), Sum1/1  "y_model"
  Sum/1 -> y_est_no_delay/1  "y_est_undelayed"

== system B4_quadcopter_model_discrete/Discrete Model - Complementary Filtering/Plant and State Estimation/Complementary Filter1 ==
  y : Inport
  y_model : Inport  Port=2
  Butterworth Lowpass 2nd Order1 : Subsystem
  Butterworth Lowpass 2nd Order2 : Subsystem
  Sum : Sum  Inputs=|++
  Sum1 : Sum  Inputs=|+-
  y_est_no_delay : Outport
  wires:
  y/1 -> Butterworth Lowpass 2nd Order1/1(In)  "y"
  Butterworth Lowpass 2nd Order1/1(Out) -> Sum/1  "y_f"
  Butterworth Lowpass 2nd Order2/1(Out) -> Sum1/2  "y_model_f"
  Sum1/1 -> Sum/2
  y_model/1 -> Butterworth Lowpass 2nd Order2/1(In), Sum1/1  "y_model"
  Sum/1 -> y_est_no_delay/1  "y_est_undelayed"

== system B4_quadcopter_model_discrete/Discrete Model - Complementary Filtering/Plant and State Estimation/Noise Acc ==
  Constant : Constant  Value=NOISE  SampleTime=sampling_time
  Merge : Merge
  Switch Case : SwitchCase
  Switch Case Action Subsystem : Subsystem  TreatAsAtomicUnit=on
  Switch Case Action Subsystem1 : Subsystem  TreatAsAtomicUnit=on
  Out : Outport
  wires:
  Switch Case/2 -> Switch Case Action Subsystem1/Action
  Merge/1 -> Out/1
  Switch Case/1 -> Switch Case Action Subsystem/Action
  Constant/1 -> Switch Case/1
  Switch Case Action Subsystem1/1(Out1) -> Merge/2
  Switch Case Action Subsystem/1(Out1) -> Merge/1

== system B4_quadcopter_model_discrete/Discrete Model - Complementary Filtering/Plant and State Estimation/Noise Gyro ==
  Constant : Constant  Value=NOISE  SampleTime=sampling_time
  Merge : Merge
  Switch Case : SwitchCase
  Switch Case Action Subsystem : Subsystem  TreatAsAtomicUnit=on
  Switch Case Action Subsystem1 : Subsystem  TreatAsAtomicUnit=on
  Out : Outport
  wires:
  Switch Case/2 -> Switch Case Action Subsystem1/Action
  Merge/1 -> Out/1
  Switch Case/1 -> Switch Case Action Subsystem/Action
  Constant/1 -> Switch Case/1
  Switch Case Action Subsystem1/1(Out1) -> Merge/2
  Switch Case Action Subsystem/1(Out1) -> Merge/1

== system B4_quadcopter_model_discrete/Discrete Model - Complementary Filtering/Plant and State Estimation/Plant Dynamics Continuous ==
  note: Attitude Calculations
  note: Rotation Matrices Calculations
  note: Position Calculations
  mass : Inport
  Force in earth frame : Inport  Port=2
  Moments in the body frame : Inport  Port=3
  Constant1 : Constant  Value=I  SampleTime=sampling_time
  Demux{,1..7} (8 alike) : Demux  Outputs=3
  Disturbance Block : Subsystem
  Divide : Product  Inputs=*/
  Integrator{2..4,12} (4 alike) : Integrator
  Invert 3x3 Matrix1 : aerolibutil/Invert  3x3 Matrix
  Matrix Multiply{1..5} (5 alike) : Product  Multiplication=Matrix(*)
  Omega_I_Omega1 : Subsystem
  Subtract : Sum
  Sum{,1..3} (4 alike) : Sum  Inputs=|++
  Transpose : Math  Operator=transpose  SaturateOnIntegerOverflow=on
  Vector Concatenate : Concatenate  NumInputs=3
  Vector Concatenate1 : Concatenate  NumInputs=3
  body_to_ground_transorm : MATLAB Function  Description=|  TreatAsAtomicUnit=on
      | This function computes the rotational matrix to pass from the body frame to the world frame. 
      | Takes as inpout the euler angles.
  euler_rates_to_pqr : MATLAB Function  TreatAsAtomicUnit=on
  g1 : Constant  Value=9.81  VectorParams1D=off
  k : Constant  Value=0  VectorParams1D=off
  pqr_to_euler_rates : MATLAB Function  TreatAsAtomicUnit=on
  wrapper : MATLAB Function  TreatAsAtomicUnit=on
  R : Outport
  T : Outport  Port=2
  R_bg : Outport  Port=3
  pqr_dot_body : Outport  Port=4
  AxAyAz_body : Outport  Port=5
  tag scope: Vx_cont=global, Vy_cont=global, Vz_cont=global, X_cont=global, Y_cont=global, Z_cont=global, p_cont=global, phi_cont=global, psi_cont=global, q_cont=global, r_cont=global, theta_cont=global, u_cont=global, ud_cont=global, v_cont=global, vd_cont=global, w_cont=global, wd_cont=global, x_cont=global, y_cont=global, z_cont=global
  wires:
  Demux/1 -> Sum/1
  Sum2/1 -> Vector Concatenate1/3
  Integrator2/1 -> Demux2/1  "Euler_angles"
  Integrator12/1 -> Demux7/1, Matrix Multiply4/2  "pqr_body"
  Divide/1 -> Subtract/2
  Matrix Multiply5/1 -> AxAyAz_body/1, Demux4/1
  mass/1 -> Divide/2
  Integrator4/1 -> Demux6/1, Matrix Multiply2/2  "xyz_earth"
  Demux2/1 -> pqr_to_euler_rates/1(Phi), euler_rates_to_pqr/1(Phi), [phi_cont], body_to_ground_transorm/1(Phi)  "Phi"
  Vector Concatenate1/1 -> Integrator12/1, pqr_dot_body/1
  Demux/2 -> Sum1/1
  Matrix Multiply3/1 -> Demux1/1
  Demux/3 -> Sum2/1
  Transpose/1 -> Matrix Multiply2/1, Matrix Multiply3/1, Matrix Multiply5/1
  k/1 -> Vector Concatenate/2, Vector Concatenate/1
  Vector Concatenate/1 -> Subtract/1
  pqr_to_euler_rates/1(T) -> T/1, Matrix Multiply4/1  "T"
  Subtract/1 -> Integrator3/1, Matrix Multiply5/2  "AxAyAz_earth"
  Integrator3/1 -> Matrix Multiply3/2, Demux5/1, Integrator4/1  "VxVyVz_earth"
  Matrix Multiply2/1 -> Demux3/1
  Force in earth frame/1 -> Divide/1
  Demux2/3 -> wrapper/1(pis_e)  "Psi"
  Sum/1 -> Vector Concatenate1/1
  Sum1/1 -> Vector Concatenate1/2
  body_to_ground_transorm/1(R_bg) -> Transpose/1, R_bg/1
  g1/1 -> Vector Concatenate/3
  Constant1/1 -> Invert 3x3 Matrix1/1, Omega_I_Omega1/2(Inertia)
  Moments in the body frame/1 -> Sum3/2
  euler_rates_to_pqr/1(R) -> R/1
  Invert 3x3 Matrix1/1 -> Matrix Multiply1/1
  Matrix Multiply1/1 -> Demux/1
  Demux1/1 -> [u_cont]
  Demux1/2 -> [v_cont]
  Demux1/3 -> [w_cont]
  Demux3/1 -> [x_cont]
  Demux3/2 -> [y_cont]
  Demux3/3 -> [z_cont]
  Demux4/1 -> [ud_cont]
  Demux4/2 -> [vd_cont]
  Demux4/3 -> [wd_cont]
  Sum3/1 -> Matrix Multiply1/2
  Omega_I_Omega1/1(Final product) -> Sum3/1
  Matrix Multiply4/1 -> Integrator2/1
  Demux2/2 -> [theta_cont], body_to_ground_transorm/2(Theta), pqr_to_euler_rates/2(Theta), euler_rates_to_pqr/2(Theta)  "Theta"
  wrapper/1(psie_w) -> [psi_cont], body_to_ground_transorm/3(Psi)  "psi"
  Demux5/1 -> [Vx_cont]
  Demux5/2 -> [Vy_cont]
  Demux5/3 -> [Vz_cont]
  Demux6/1 -> [X_cont]
  Demux6/2 -> [Y_cont]
  Demux6/3 -> [Z_cont]
  Demux7/1 -> [p_cont]
  Demux7/2 -> [q_cont]
  Demux7/3 -> [r_cont]

== system B4_quadcopter_model_discrete/Discrete Model - Complementary Filtering/Plant and State Estimation/Subsystem1 ==
  Add : Sum
  Constant4 : Constant  Value=K_t  SampleTime=sampling_time
  Forces due to thrust : MATLAB Function  TreatAsAtomicUnit=on
  Gain : Gain  Gain=1/m
  Subtract : Sum
  Terminator : Terminator
  Vector Concatenate : Concatenate  NumInputs=3
  g1 : Constant  Value=9.81  VectorParams1D=off
  k : Constant  Value=0  VectorParams1D=off
  y_model : Outport
  wires:
  Forces due to thrust/1(F_t_e) -> Add/2  "thrust_earth"
  Constant4/1 -> Forces due to thrust/6(K_t)
  [R_bg_discr] -> Forces due to thrust/5(R_bg)
  [omega_1_f] -> Forces due to thrust/1(omega_1)
  [omega_2_f] -> Forces due to thrust/2(omega_2)
  [omega_3_f] -> Forces due to thrust/3(omega_3)
  [omega_4_f] -> Forces due to thrust/4(omega_4)
  Gain/1 -> Subtract/2
  Vector Concatenate/1 -> Subtract/1
  k/1 -> Vector Concatenate/2, Vector Concatenate/1
  g1/1 -> Vector Concatenate/3
  Subtract/1 -> y_model/1  "AxAyAz_earth"
  Add/1 -> Gain/1
  Forces due to thrust/2(F_t_b) -> Terminator/1  "thrust_body"

== system B4_quadcopter_model_discrete/Discrete Model - Doublet/Continuous Actuator Dynamics/Butterworth Lowpass 2nd Order1 ==
  In : Inport
  Constant : Constant  Value=FILTER  SampleTime=sampling_time
  Merge : Merge
  Switch Case : SwitchCase
  Switch Case Action Subsystem : Subsystem  TreatAsAtomicUnit=on
  Switch Case Action Subsystem1 : Subsystem  TreatAsAtomicUnit=on
  Out : Outport
  wires:
  Merge/1 -> Out/1
  Switch Case Action Subsystem/1(Out1) -> Merge/1
  Constant/1 -> Switch Case/1
  Switch Case Action Subsystem1/1(Out1) -> Merge/2
  Switch Case/2 -> Switch Case Action Subsystem1/Action
  In/1 -> Switch Case Action Subsystem/1(In1), Switch Case Action Subsystem1/1(In1)
  Switch Case/1 -> Switch Case Action Subsystem/Action

== system B4_quadcopter_model_discrete/Discrete Model - Doublet/Discrete INDI Controller Cascaded/ERROR CONTROLLER ATTITUDE ==
  p_ref : Inport
  q_ref : Inport  Port=2
  r_ref : Inport  Port=3
  phi_ref : Inport  Port=4
  theta_ref : Inport  Port=5
  psi_ref : Inport  Port=6
  Abs : Abs
  Add : Sum  Inputs=+++
  Add1 : Sum  Inputs=+++
  Add2 : Sum  Inputs=+++
  Cumulative Sum : dspmathops/Cumulative Sum  dim=Channels (running sum)  InputProcessing=Columns as channels (frame based)  reset_popup=None  roundingMode=Floor  overflowMode=off  outputDataTypeStr=Inherit: Same as accumulator  outputMin=[]  outputMax=[]  outputLastDataTypeStr=Inherit: Same as accumulator
  Display : Display
  Display1 : Display
  Gain1 : Gain  Gain=K_ec_d_p
  Gain2 : Gain  Gain=K_ec_p
  Gain4 : Gain  Gain=K_ec_d_q
  Gain5 : Gain  Gain=K_ec_q
  Gain7 : Gain  Gain=K_ec_d_r
  Gain8 : Gain  Gain=K_ec_r
  MATLAB Function1 : MATLAB Function  TreatAsAtomicUnit=on
  Mean : dspstat3/Mean  run=off  InputProcessing=Columns as channels (frame based)  reset_popup=None  directionMode=Each column  dimension=1  roiEnable=off  roiType=Rectangles  roiPortion=Entire ROI  roiOutput=Individual statistics for each ROI  roiFlag=off  roundingMode=Floor  overflowMode=off  outputDataTypeStr=Inherit: Same as accumulator  outputMin=[]  outputMax=[]  outputLastDataTypeStr=Inherit: Same as accumulator
  Sum{1..2,4..5,7..8} (6 alike) : Sum  Inputs=|+-
  pd_ec : Outport
  qd_ec : Outport  Port=2
  rd_ec : Outport  Port=3
  wires:
  p_ref/1 -> Sum1/1
  Add/1 -> pd_ec/1
  [p] -> Sum1/2
  [phi] -> Sum2/2
  phi_ref/1 -> Sum2/1
  Sum1/1 -> Gain1/1  "p_err"
  Sum2/1 -> Gain2/1  "phi_err"
  Gain1/1 -> Add/2
  Gain2/1 -> Add/3
  Sum4/1 -> Gain4/1  "q_err"
  Sum5/1 -> Abs/1, Gain5/1  "theta_err"
  Gain4/1 -> Add1/2
  Gain5/1 -> Add1/3
  theta_ref/1 -> Sum5/1
  [theta] -> Sum5/2
  [q] -> Sum4/2
  q_ref/1 -> Sum4/1
  Add1/1 -> qd_ec/1
  Sum7/1 -> Gain7/1  "r_err"
  MATLAB Function1/1(psie_w) -> Gain8/1  "psi_err"
  Gain7/1 -> Add2/2
  Gain8/1 -> Add2/3
  psi_ref/1 -> Sum8/1
  [psi] -> Sum8/2
  [r] -> Sum7/2
  r_ref/1 -> Sum7/1
  Add2/1 -> rd_ec/1
  Sum8/1 -> MATLAB Function1/1(pis_e)
  Cumulative Sum/1 -> Display/1
  Mean/1 -> Display1/1
  Abs/1 -> Mean/1, Cumulative Sum/1  "theta_err_abs"

== system B4_quadcopter_model_discrete/Discrete Model - Doublet/Discrete INDI Controller Cascaded/ERROR CONTROLLER VELOCITY ==
  Vx_ref : Inport
  Vy_ref : Inport  Port=2
  Vz_ref : Inport  Port=3
  Discrete-Time Integrator : DiscreteIntegrator  SampleTime=-1  ICPrevOutput=DiscIntNeverNeededParam  ICPrevScaledInput=DiscIntNeverNeededParam
  Discrete-Time Integrator1 : DiscreteIntegrator  SampleTime=-1  ICPrevOutput=DiscIntNeverNeededParam  ICPrevScaledInput=DiscIntNeverNeededParam
  Discrete-Time Integrator2 : DiscreteIntegrator  SampleTime=-1  ICPrevOutput=DiscIntNeverNeededParam  ICPrevScaledInput=DiscIntNeverNeededParam
  Gain{,1..5} (6 alike) : Gain  Gain=5
  Scope : Scope  NumInputPorts=2
  Sum : Sum  Inputs=|+-
  Sum1 : Sum  Inputs=|++
  Sum2 : Sum  Inputs=|++
  Sum3 : Sum  Inputs=|+-
  Sum4 : Sum  Inputs=|++
  Sum6 : Sum  Inputs=|+-
  Ax_ec : Outport
  Ay_ec : Outport  Port=2
  Az_ec : Outport  Port=3
  wires:
  [Vz] -> Sum6/2
  Gain3/1 -> Sum2/2
  Gain1/1 -> Sum1/2
  Sum1/1 -> Ax_ec/1
  Gain2/1 -> Sum2/1
  Discrete-Time Integrator/1 -> Gain5/1
  Sum2/1 -> Ay_ec/1
  Vy_ref/1 -> Sum3/1
  Gain4/1 -> Sum4/1
  Discrete-Time Integrator1/1 -> Gain3/1
  Gain/1 -> Sum1/1
  Vx_ref/1 -> Sum/1
  Sum6/1 -> Discrete-Time Integrator/1, Gain4/1  "Vz_error"
  [Vy] -> Sum3/2
  Vz_ref/1 -> Sum6/1
  Sum/1 -> Discrete-Time Integrator2/1, Scope/1, Gain/1  "Vx_error"
  Sum4/1 -> Az_ec/1
  Gain5/1 -> Sum4/2
  [Vx] -> Sum/2
  Sum3/1 -> Discrete-Time Integrator1/1, Gain2/1  "Vy_error"
  Discrete-Time Integrator2/1 -> Scope/2, Gain1/1

== system B4_quadcopter_model_discrete/Discrete Model - Doublet/Discrete INDI Controller Cascaded/INTERNAL REFERENCE MODEL ATTITUDE ==
  phi_cmd : Inport
  theta_cmd : Inport  Port=2
  psi_cmd : Inport  Port=3
  Discrete-Time Integrator{,1..5} (6 alike) : DiscreteIntegrator  SampleTime=-1  ICPrevOutput=DiscIntNeverNeededParam  ICPrevScaledInput=DiscIntNeverNeededParam
  Gain4 : Gain  Gain=K_p_d
  Gain5 : Gain  Gain=K_q_d
  Gain6 : Gain  Gain=K_r_d
  Gain7 : Gain  Gain=K_p
  Gain8 : Gain  Gain=K_q
  Gain9 : Gain  Gain=K_r
  MATLAB Function1 : MATLAB Function  TreatAsAtomicUnit=on
  Sum{1,11,16,20..22} (6 alike) : Sum  Inputs=|+-
  body rates to euler rates : Subsystem
  euler rates to body rates : Subsystem
  pd_ref : Outport
  qd_ref : Outport  Port=2
  rd_ref : Outport  Port=3
  p_ref : Outport  Port=4
  q_ref : Outport  Port=5
  r_ref : Outport  Port=6
  phi_ref : Outport  Port=7
  theta_ref : Outport  Port=8
  psi_ref : Outport  Port=9
  wires:
  Discrete-Time Integrator2/1 -> theta_ref/1, Sum11/2  "theta_ref"
  Gain6/1 -> Discrete-Time Integrator5/1, rd_ref/1  "rd_ref"
  Discrete-Time Integrator/1 -> body rates to euler rates/1(p), p_ref/1, Sum21/2  "p_ref"
  Discrete-Time Integrator5/1 -> body rates to euler rates/3(r), r_ref/1, Sum22/2  "r_ref"
  Discrete-Time Integrator4/1 -> body rates to euler rates/2(q), q_ref/1, Sum16/2  "q_ref"
  Gain5/1 -> Discrete-Time Integrator4/1, qd_ref/1  "qd_ref"
  Sum21/1 -> Gain4/1
  Sum11/1 -> Gain8/1
  Sum22/1 -> Gain6/1
  Sum16/1 -> Gain5/1
  Discrete-Time Integrator1/1 -> phi_ref/1, Sum20/2  "phi_ref"
  Sum20/1 -> Gain7/1
  Gain4/1 -> Discrete-Time Integrator/1, pd_ref/1  "pd_ref"
  phi_cmd/1 -> Sum20/1
  theta_cmd/1 -> Sum11/1
  psi_cmd/1 -> Sum1/1
  Discrete-Time Integrator3/1 -> psi_ref/1, Sum1/2  "psi_ref"
  Sum1/1 -> MATLAB Function1/1(pis_e)
  euler rates to body rates/2(q) -> Sum16/1
  euler rates to body rates/1(p) -> Sum21/1
  euler rates to body rates/3(r) -> Sum22/1
  Gain9/1 -> euler rates to body rates/3(psi_dot)
  Gain8/1 -> euler rates to body rates/2(theta_dot)
  Gain7/1 -> euler rates to body rates/1(phi_dot)
  body rates to euler rates/1(phi_dot) -> Discrete-Time Integrator1/1
  body rates to euler rates/2(theta_dot) -> Discrete-Time Integrator2/1
  body rates to euler rates/3(psi_dot) -> Discrete-Time Integrator3/1
  MATLAB Function1/1(psie_w) -> Gain9/1
